simulink model "PowerFactorMeter_R2019b"  (R2019b)
settings: Solver=VariableStepAuto  StartTime=0.0  StopTime=0.1  RelTol=1e-3
libraries: powerlib x6, eePowerMeasurement x1
settings Model: Creator=FAST  LastModifiedBy=FAST

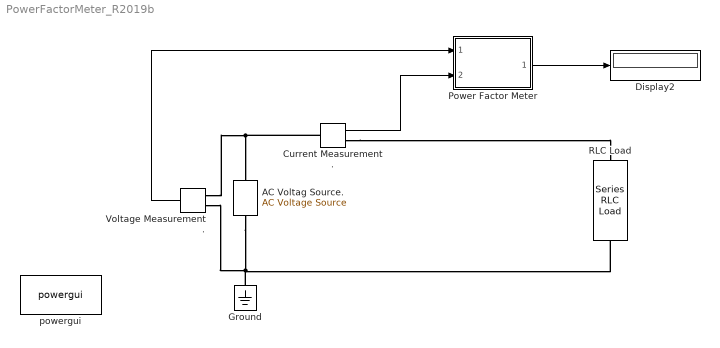
== system PowerFactorMeter_R2019b ==
  " RLC Load" : powerlib/Elements/Series RLC Load  LConnTagsString=a  RConnTagsString=__new0  NominalVoltage=1000  NominalFrequency=60  ActivePower=10e3  InductivePower=5000  CapacitivePower=3000  Setx0=off  InitialVoltage=0  SetiL0=off  InitialCurrent=0  Measurements=None  LoadType=constant Z
      settings: SourceProductName=Simscape Electrical
  AC Voltag Source. : powerlib/Electrical Sources/AC Voltage Source  Amplitude=100  Phase=0  Frequency=60  SampleTime=0  Measurements=None  BusType=swing  Pref=10e3  Qref=0  Qmin=-inf  Qmax=+inf
      settings: SourceProductName=Simscape Electrical
  Current Measurement. : powerlib/Measurements/Current Measurement  PhasorSimulation=off  OutputType=Complex  PSBequivalent=0
      settings: SourceProductName=Simscape Electrical
  Display2 : Display
  Ground : powerlib/Elements/Ground  LConnTagsString=a
      settings: SourceProductName=Simscape Electrical
  Power Factor Meter : Subsystem  mask{F=60}
      mask prompts: F "Frequency"
      mask help:
      | Power Factor meter
      | __________________________________________________
      | This block calculates power factor measurement by implementing the following:
      | S^2=P^2+Q^2
      | S=sqrt(S^2)
      | cos(theta)=Q/S
      | where:
      | 	P=Real power
      | 	Q= Reactive power
      | 	S=Apparent power
      | 	PF=cos(theta)
      |
      | In this block P and Q are measured by using power measurement block which is a built in  block in SIMULINK
  Voltage Measurement. : powerlib/Measurements/Voltage Measurement  PhasorSimulation=off  OutputType=Complex  PSBequivalent=0
      settings: SourceProductName=Simscape Electrical
  powergui : powerlib/powergui  Priority=1  SimulationMode=Continuous  SampleTime=50e-6  frequency=60  Iterations=50  frequencyindice=60  Pbase=100e6  ErrMax=1e-4  UnitsV=kV  UnitsW=MW  buscounter=0  FunctionMessages=off  echomessages=off  EnableUseOfTLC=off  CurrentSourceSwitches=off  DisableSnubberDevices=off  DisableRonSwitches=off  DisableVfSwitches=off  DisplayEquations=off  AutomaticDiscreteSolvers=off  SolverType=Tustin/Backward Euler (TBE)  Interpol=off  ExternalGateDelay=off  methode=off  Ts=100  x0status=blocks  SPID=on  SwTol=0  HookPort=off  NonlinearTolerance=1e-4  nMaxIteration=100  ContinueOnMaxIteration=off  RestoreLinks=warning  ResistiveCurrentMeasurement=off  Frange=[0:2:500]  Ylog=off  Xlog=on  ShowGrid=off  save=off  variable=ZData  structure=0  ZoomFFT=off  StartTime=0.0  cycles=1  DisplayStyle=1  fundamental=60  FreqAxis=off  MaxFrequency=1000  frequencyindicesteady=1  RmsSteady=1  display=off
      settings: SourceProductName=Simscape Electrical
  wires:
  Current Measurement./1 -> Power Factor Meter/2(Current)
  Power Factor Meter/1(power factor) -> Display2/1
  Voltage Measurement./1 -> Power Factor Meter/1(Voltage)
  connections:
  AC Voltag Source./LConn1 -- Voltage Measurement./LConn2 -- " RLC Load"/RConn1 -- Ground/LConn1
  Current Measurement./LConn1 -- AC Voltag Source./RConn1 -- Voltage Measurement./LConn1
  Current Measurement./RConn1 -- " RLC Load"/LConn1

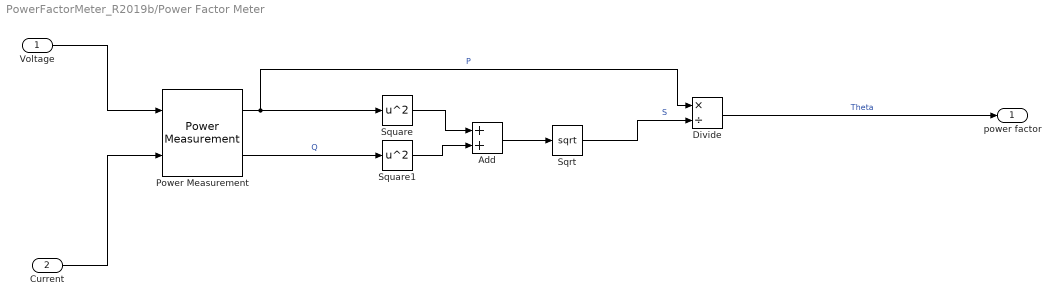
== system PowerFactorMeter_R2019b/Power Factor Meter ==
  Voltage : Inport
  Current : Inport  Port=2
  Add : Sum
  Divide : Product  Inputs=*/
  Power Measurement : eePowerMeasurement/Power Measurement  LabelModeActiveChoice=Continuous  F=F  K=[1]  Ts=0
      settings: SourceProductName=Simscape Electrical  SourceProductBaseCode=PS
  Sqrt : Sqrt  SaturateOnIntegerOverflow=on
  Square : Math  Operator=square  SaturateOnIntegerOverflow=on
  Square1 : Math  Operator=square  SaturateOnIntegerOverflow=on
  power factor : Outport  VectorParamsAs1DForOutWhenUnconnected=off
  wires:
  Add/1 -> Sqrt/1
  Current/1 -> Power Measurement/2
  Square/1 -> Add/1
  Sqrt/1 -> Divide/2  "S"
  Power Measurement/1 -> Square/1, Divide/1  "P"
  Voltage/1 -> Power Measurement/1
  Power Measurement/2 -> Square1/1  "Q"
  Square1/1 -> Add/2
  Divide/1 -> power factor/1  "Theta"
